simulink model "BESSmodel_EMT_2019a"  (R2019a)
settings: Solver=VariableStepAuto  SolverName=ode4  StartTime=0.0  StopTime=10  FixedStep=100e-6  RelTol=1e-3
undefined symbols (not defined in the file): D11, Delta, Ion, Lithium
libraries: powerlib x24, powerlib_meascontrol x15, simulink x9, eeGeneralControl x8, electricdrivelib x1
(part 2 of 2)

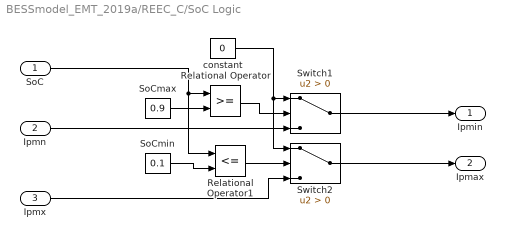
== system BESSmodel_EMT_2019a/REEC_C/SoC Logic ==
  SoC : Inport
  Ipmn : Inport  Port=2
  Ipmx : Inport  Port=3
  Relational Operator : RelationalOperator  OutDataTypeStr=boolean  RndMeth=Simplest
  Relational Operator1 : RelationalOperator  Operator=<=  OutDataTypeStr=boolean  RndMeth=Simplest
  SoCmax : Constant  Value=0.9
  SoCmin : Constant  Value=0.1
  Switch1 : Switch  Criteria=u2 > Threshold
  Switch2 : Switch  Criteria=u2 > Threshold
  constant : Constant  Value=0
  Ipmin : Outport
  Ipmax : Outport  Port=2
  wires:
  SoC/1 -> Relational Operator/1, Relational Operator1/1
  Ipmx/1 -> Switch2/3
  constant/1 -> Switch2/1, Switch1/1
  Switch1/1 -> Ipmin/1
  Relational Operator1/1 -> Switch2/2
  Relational Operator/1 -> Switch1/2
  SoCmax/1 -> Relational Operator/2
  SoCmin/1 -> Relational Operator1/2
  Ipmn/1 -> Switch1/3
  Switch2/1 -> Ipmax/1

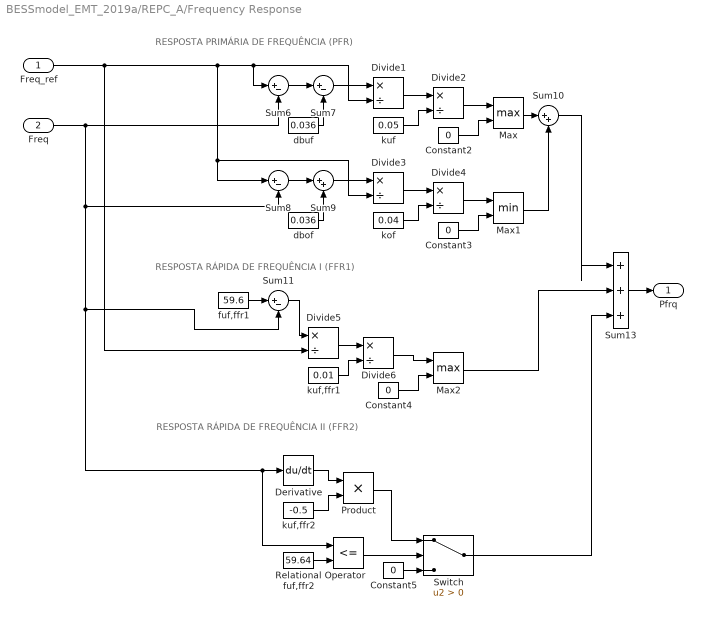
== system BESSmodel_EMT_2019a/REPC_A/Frequency Response ==
  note: RESPOSTA RÁPIDA DE FREQUÊNCIA II (FFR2)
  note: RESPOSTA RÁPIDA DE FREQUÊNCIA I (FFR1)
  note: RESPOSTA PRIMÁRIA DE FREQUÊNCIA (PFR)
  Freq_ref : Inport
  Freq : Inport  Port=2
  Constant{2..5} (4 alike) : Constant  Value=0
  Derivative : Derivative
  Divide{1..6} (6 alike) : Product  Inputs=*/
  Max : MinMax  Function=max  Inputs=2
  Max1 : MinMax  Inputs=2
  Max2 : MinMax  Function=max  Inputs=2
  Product : Product
  Relational Operator : RelationalOperator  Operator=<=  OutDataTypeStr=boolean  RndMeth=Simplest
  Sum10 : Sum  Inputs=|++
  Sum{6..8,11} (4 alike) : Sum  Inputs=|+-
  Sum13 : Sum  Inputs=|+++
  Sum9 : Sum  Inputs=|++
  Switch : Switch  Criteria=u2 > Threshold
  dbof : Constant  Value=0.036
  dbuf : Constant  Value=0.036
  fuf,ffr1 : Constant  Value=59.6
  fuf,ffr2 : Constant  Value=59.64
  kof : Constant  Value=0.04
  kuf : Constant  Value=0.05
  kuf,ffr1 : Constant  Value=0.01
  kuf,ffr2 : Constant  Value=-0.5
  Pfrq : Outport
  wires:
  Sum10/1 -> Sum13/1
  Max/1 -> Sum10/1
  Freq/1 -> Sum6/2, Sum8/2, Sum11/2, Relational Operator/1, Derivative/1
  Freq_ref/1 -> Divide3/2, Sum8/1, Sum6/1, Divide1/2, Divide5/2
  Sum11/1 -> Divide5/1
  Sum9/1 -> Divide3/1
  Sum8/1 -> Sum9/1
  kuf,ffr2/1 -> Product/2
  Divide5/1 -> Divide6/1
  kuf/1 -> Divide2/2
  Constant3/1 -> Max1/2
  dbuf/1 -> Sum7/2
  dbof/1 -> Sum9/2
  kof/1 -> Divide4/2
  Divide4/1 -> Max1/1
  Max2/1 -> Sum13/2
  Derivative/1 -> Product/1
  Constant5/1 -> Switch/3
  Divide1/1 -> Divide2/1
  Product/1 -> Switch/1
  Divide2/1 -> Max/1
  fuf,ffr1/1 -> Sum11/1
  Sum13/1 -> Pfrq/1
  kuf,ffr1/1 -> Divide6/2
  Sum7/1 -> Divide1/1
  Constant2/1 -> Max/2
  Constant4/1 -> Max2/2
  Divide3/1 -> Divide4/1
  Sum6/1 -> Sum7/1
  Switch/1 -> Sum13/3
  Max1/1 -> Sum10/2
  fuf,ffr2/1 -> Relational Operator/2
  Relational Operator/1 -> Switch/2
  Divide6/1 -> Max2/1

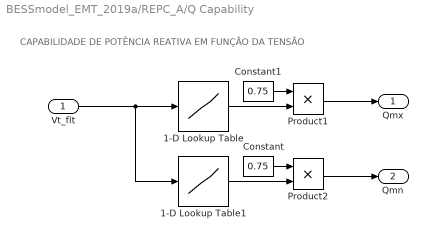
== system BESSmodel_EMT_2019a/REPC_A/Q Capability ==
  note: CAPABILIDADE DE POTÊNCIA REATIVA EM FUNÇÃO DA TENSÃO
  Vt_flt : Inport
  1-D Lookup Table : Lookup_n-D  NumberOfTableDimensions=1  BreakpointsForDimension1=[0.9;0.95;1.03;1.05]  Table=[0.7;1;1;0]  InternalRulePriority=Speed  RndMeth=Simplest  InputSameDT=on
  1-D Lookup Table1 : Lookup_n-D  NumberOfTableDimensions=1  BreakpointsForDimension1=[0.95;0.99;1.05;1.0501]  Table=[0;-1;-1;0]  InternalRulePriority=Speed  RndMeth=Simplest  InputSameDT=on
  Constant : Constant  Value=0.75
  Constant1 : Constant  Value=0.75
  Product1 : Product
  Product2 : Product
  Qmx : Outport
  Qmn : Outport  Port=2
  wires:
  Constant1/1 -> Product1/1
  1-D Lookup Table/1 -> Product1/2
  1-D Lookup Table1/1 -> Product2/2
  Vt_flt/1 -> 1-D Lookup Table1/1, 1-D Lookup Table/1
  Constant/1 -> Product2/1
  Product2/1 -> Qmn/1
  Product1/1 -> Qmx/1
